simulink model "Gravity_Compensation"  (R2019a)
settings: Solver=FixedStepAuto  StartTime=0.0  StopTime=inf  RelTol=1e-3  EnableMultiTasking=on
libraries: eeGeneralControl x2, cm_custom x2
settings Model: SimulationMode=external  Creator=Ng Wee Shen  LastModifiedBy=rng
settings SolverCC: PositivePriorityOrder=on  AutoInsertRateTranBlk=on
settings DataIOCC: ReturnWorkspaceOutputs=off
settings OptimizationCC: EnhancedBackFolding=on  PassReuseOutputArgsAs=Individual arguments  MaxStackSize=64  OptimizeBlockOrder=speed  DifferentSizesBufferReuse=on
settings DebuggingCC: TimeAdjustmentMsg=warning  SingleTaskRateTransMsg=warning  ParameterTunabilityLossMsg=error  SFcnCompatibilityMsg=warning  ArithmeticOperatorsInVariantConditions=warning
settings HardwareCC: ProdBitPerPointer=32  ProdBitPerSizeT=32  ProdBitPerPtrDiffT=32  ProdLargestAtomicInteger=Long  ProdLargestAtomicFloat=Double  ProdWordSize=32  ProdHWDeviceType=ARM Compatible->ARM Cortex
settings SFSimCC: MATLABDynamicMemAlloc=off
settings RTWCC: SystemTargetFile=ert.tlc  HardwareBoard=Raspberry Pi  TLCOptions="-aInlineSetEventsForThisBaseRateFcn=TLC_FALSE -aSuppressMultiTaskScheduler=TLC_FALSE  -aRateBasedStepFcn=0"  TemplateMakefile=ert_default_tmf  Toolchain=GNU GCC Raspberry Pi  BuildConfiguration=Specify  IncludeHyperlinkInReport=on  TargetLang=C++
settings CodeAppCC: ForceParamTrailComments=on  IgnoreCustomStorageClasses=off  OperatorAnnotations=on  SimulinkDataObjDesc=on  SFDataObjDesc=on  InsertBlockDesc=on
settings ERTTargetCC: TargetLangStandard=C++03 (ISO)  SupportContinuousTime=on  SupportVariableSizeSignals=on  ExtMode=on  ExtModeMexArgs='192.168.0.173' 1 17725

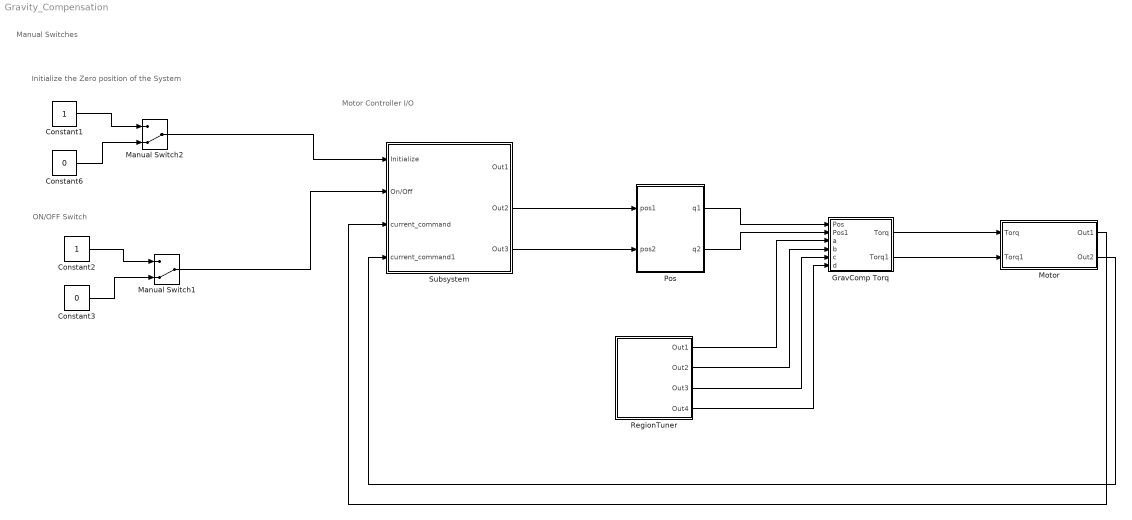
== system Gravity_Compensation ==
  note: Motor Controller I/O
  note: Manual Switches
  note: ON/OFF Switch
  note: Initialize the Zero position of the System
  Constant1 : Constant
  Constant2 : Constant
  Constant3 : Constant  Value=0
  Constant6 : Constant  Value=0
  GravComp Torq : MATLAB Function  TreatAsAtomicUnit=on
  Manual Switch1 : ManualSwitch  CurrentSetting=0
  Manual Switch2 : ManualSwitch  CurrentSetting=0
  Motor : Subsystem
  Pos : Subsystem
  RegionTuner : Subsystem
  Subsystem : Subsystem
  wires:
  Constant1/1 -> Manual Switch2/1
  Constant6/1 -> Manual Switch2/2
  Manual Switch2/1 -> Subsystem/1(Initialize)
  Subsystem/2(Out2) -> Pos/1(pos1)
  Subsystem/3(Out3) -> Pos/2(pos2)
  Constant2/1 -> Manual Switch1/1
  Constant3/1 -> Manual Switch1/2
  Manual Switch1/1 -> Subsystem/2(On/Off)
  GravComp Torq/1(Torq) -> Motor/1(Torq)
  GravComp Torq/2(Torq1) -> Motor/2(Torq1)
  Pos/1(q1) -> GravComp Torq/1(Pos)
  Pos/2(q2) -> GravComp Torq/2(Pos1)
  RegionTuner/1(Out1) -> GravComp Torq/3(a)
  RegionTuner/2(Out2) -> GravComp Torq/4(b)
  RegionTuner/3(Out3) -> GravComp Torq/5(c)
  RegionTuner/4(Out4) -> GravComp Torq/6(d)
  Motor/2(Out2) -> Subsystem/4(current_command1)
  Motor/1(Out1) -> Subsystem/3(current_command)

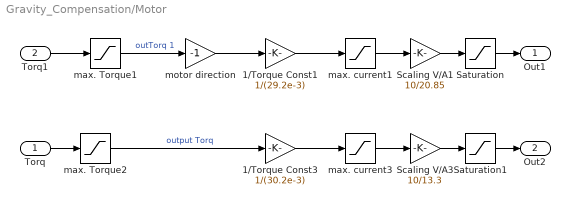
== system Gravity_Compensation/Motor ==
  Torq : Inport
  Torq1 : Inport  Port=2
  1/Torque Const1 : Gain  Gain=1/(29.2e-3)  OutDataTypeStr=Inherit: Same as input
  1/Torque Const3 : Gain  Gain=1/(30.2e-3)  OutDataTypeStr=Inherit: Same as input
  Saturation : Saturate  UpperLimit=9.95  LowerLimit=-9.95
  Saturation1 : Saturate  UpperLimit=9.95  LowerLimit=-9.95
  Scaling V/A1 : Gain  Gain=10/20.85  OutDataTypeStr=Inherit: Same as input
  Scaling V/A3 : Gain  Gain=10/13.3  OutDataTypeStr=Inherit: Same as input
  max. Torque1 : Saturate  UpperLimit=0.10  LowerLimit=-0.10
  max. Torque2 : Saturate  UpperLimit=0.05  LowerLimit=-0.05
  max. current1 : Saturate  UpperLimit=6  LowerLimit=-6
  max. current3 : Saturate  UpperLimit=6  LowerLimit=-6
  motor direction : Gain  Gain=-1  OutDataTypeStr=Inherit: Same as input
  Out1 : Outport
  Out2 : Outport  Port=2
  wires:
  max. current3/1 -> Scaling V/A3/1
  Scaling V/A3/1 -> Saturation1/1
  max. Torque2/1 -> 1/Torque Const3/1  "output Torq"
  Torq/1 -> max. Torque2/1
  1/Torque Const3/1 -> max. current3/1
  1/Torque Const1/1 -> max. current1/1
  max. current1/1 -> Scaling V/A1/1
  motor direction/1 -> 1/Torque Const1/1
  max. Torque1/1 -> motor direction/1  "outTorq 1"
  Scaling V/A1/1 -> Saturation/1
  Torq1/1 -> max. Torque1/1
  Saturation1/1 -> Out2/1
  Saturation/1 -> Out1/1

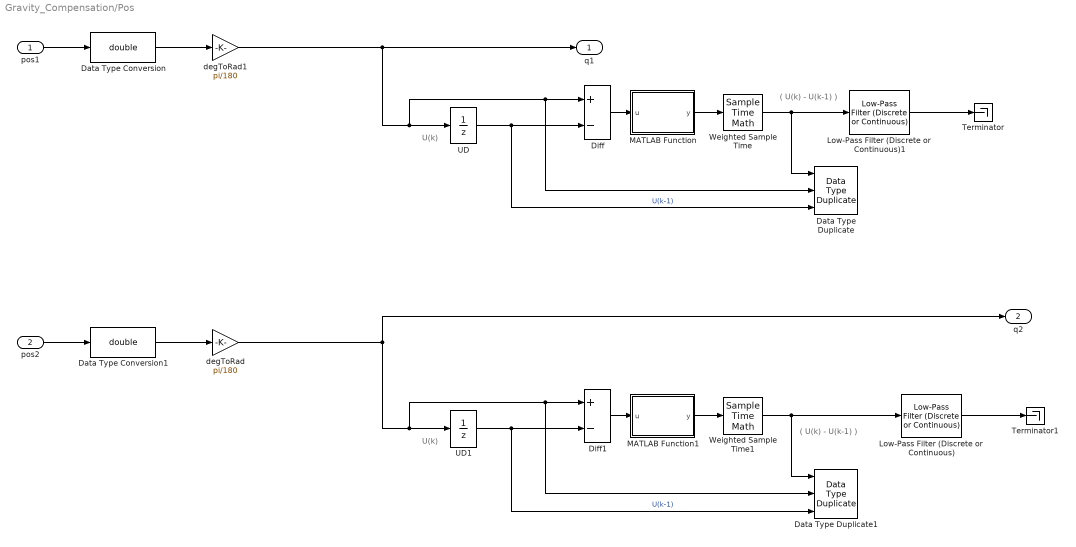
== system Gravity_Compensation/Pos ==
  note: ( U(k) - U(k-1) )
  note: U(k)
  note: U(k)
  note: ( U(k) - U(k-1) )
  pos1 : Inport
  pos2 : Inport  Port=2
  Data Type Duplicate : DataTypeDuplicate  DisableCoverage=on  NumInputPorts=3
  Data Type Duplicate1 : DataTypeDuplicate  DisableCoverage=on  NumInputPorts=3
  Data Type Conversion : DataTypeConversion  OutDataTypeStr=double
  Data Type Conversion1 : DataTypeConversion  OutDataTypeStr=double
  Diff : Sum  Description=Add in CPU  Inputs=+-
  Diff1 : Sum  Description=Add in CPU  Inputs=+-
  Low-Pass Filter (Discrete or Continuous) : eeGeneralControl/Low-Pass Filter (Discrete or Continuous)  K=1  T=0.01  B=inf  A=-inf  Ts=-1
      settings: SourceProductName=Simscape Electrical
  Low-Pass Filter (Discrete or Continuous)1 : eeGeneralControl/Low-Pass Filter (Discrete or Continuous)  K=1  T=0.01  B=inf  A=-inf  Ts=-1
      settings: SourceProductName=Simscape Electrical
  MATLAB Function : MATLAB Function  TreatAsAtomicUnit=on
  MATLAB Function1 : MATLAB Function  TreatAsAtomicUnit=on
  Terminator : Terminator
  Terminator1 : Terminator
  UD : UnitDelay  Description=Store in Global RAM  DisableCoverage=on  SampleTime=-1  HasFrameUpgradeWarning=on
  UD1 : UnitDelay  Description=Store in Global RAM  DisableCoverage=on  SampleTime=-1  HasFrameUpgradeWarning=on
  Weighted Sample Time : SampleTimeMath  TsampMathOp=/
  Weighted Sample Time1 : SampleTimeMath  TsampMathOp=/
  degToRad : Gain  Gain=pi/180
  degToRad1 : Gain  Gain=pi/180
  q1 : Outport
  q2 : Outport  Port=2
  wires:
  pos2/1 -> Data Type Conversion1/1
  pos1/1 -> Data Type Conversion/1
  Data Type Conversion1/1 -> degToRad/1
  Data Type Conversion/1 -> degToRad1/1
  Diff/1 -> MATLAB Function/1(u)
  UD/1 -> Diff/2, Data Type Duplicate/3  "U(k-1)"
  MATLAB Function/1(y) -> Weighted Sample Time/1
  Weighted Sample Time/1 -> Data Type Duplicate/1, Low-Pass Filter (Discrete or Continuous)1/1
  UD1/1 -> Diff1/2, Data Type Duplicate1/3  "U(k-1)"
  Diff1/1 -> MATLAB Function1/1(u)
  MATLAB Function1/1(y) -> Weighted Sample Time1/1
  Weighted Sample Time1/1 -> Data Type Duplicate1/1, Low-Pass Filter (Discrete or Continuous)/1
  degToRad1/1 -> q1/1, UD/1, Diff/1, Data Type Duplicate/2
  degToRad/1 -> q2/1, UD1/1, Diff1/1, Data Type Duplicate1/2
  Low-Pass Filter (Discrete or Continuous)1/1 -> Terminator/1
  Low-Pass Filter (Discrete or Continuous)/1 -> Terminator1/1

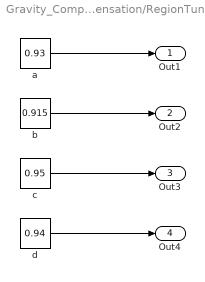
== system Gravity_Compensation/RegionTuner ==
  a : Constant  Value=0.93
  b : Constant  Value=0.915
  c : Constant  Value=0.95
  d : Constant  Value=0.94
  Out1 : Outport
  Out2 : Outport  Port=2
  Out3 : Outport  Port=3
  Out4 : Outport  Port=4
  wires:
  d/1 -> Out4/1
  b/1 -> Out2/1
  c/1 -> Out3/1
  a/1 -> Out1/1

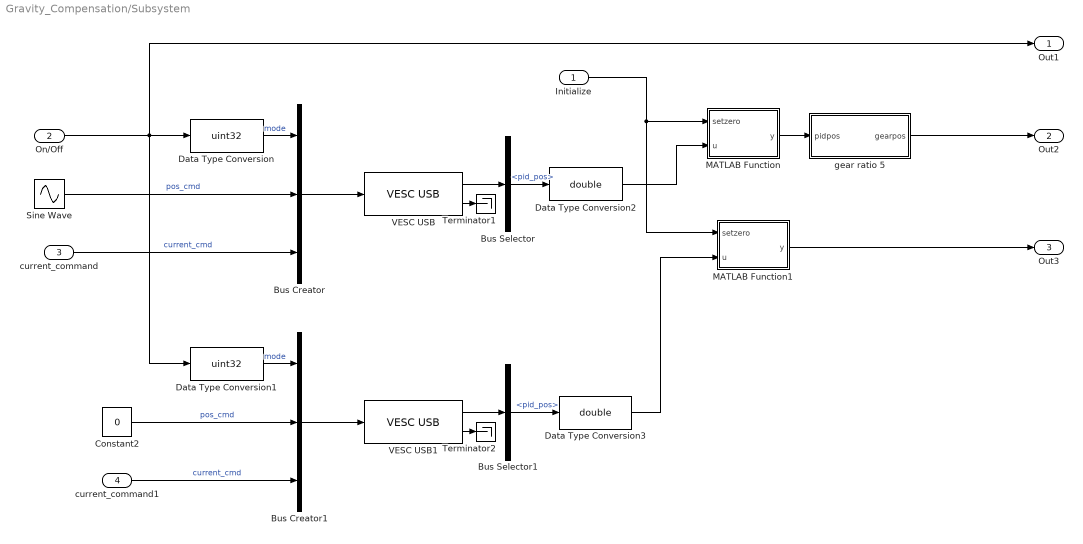
== system Gravity_Compensation/Subsystem ==
  Initialize : Inport
  On/Off : Inport  Port=2
  current_command : Inport  Port=3
  current_command1 : Inport  Port=4
  Bus Creator : BusCreator  Inputs=3
  Bus Creator1 : BusCreator  Inputs=3
  Bus Selector : BusSelector  OutputSignals=pid_pos
  Bus Selector1 : BusSelector  OutputSignals=pid_pos
  Constant2 : Constant  Value=0
  Data Type Conversion : DataTypeConversion  OutDataTypeStr=uint32
  Data Type Conversion1 : DataTypeConversion  OutDataTypeStr=uint32
  Data Type Conversion2 : DataTypeConversion  OutDataTypeStr=double
  Data Type Conversion3 : DataTypeConversion  OutDataTypeStr=double
  MATLAB Function : MATLAB Function  TreatAsAtomicUnit=on
  MATLAB Function1 : MATLAB Function  TreatAsAtomicUnit=on
  Sine Wave : Sin  Amplitude=150  Bias=10  SampleTime=0
  Terminator1 : Terminator
  Terminator2 : Terminator
  VESC USB : cm_custom/VESC USB  PAR_VESC_DEV='/dev/USB_VESC2'  POS_KP=0.03  POS_KI=0  POS_KD=0.0004  POS_KD_FIL=0.2  POS_DIV=1  CURR_MAX=6  CURR_MIN=-6  CURR_IN_MAX=99  CURR_IN_MIN=-60  CURR_ABS_MAX=130  PAR_SMPLT=0.001
      settings: SourceProductName=cm custom
  VESC USB1 : cm_custom/VESC USB  PAR_VESC_DEV='/dev/USB_VESC1'  POS_KP=0.001  POS_KI=0  POS_KD=0.001  POS_KD_FIL=0.2  POS_DIV=1  CURR_MAX=20  CURR_MIN=-20  CURR_IN_MAX=20  CURR_IN_MIN=-20  CURR_ABS_MAX=20  PAR_SMPLT=0.001
      settings: SourceProductName=cm custom
  gear ratio 5 : Subsystem
  Out1 : Outport
  Out2 : Outport  Port=2
  Out3 : Outport  Port=3
  wires:
  Bus Selector1/1 -> Data Type Conversion3/1  "<pid_pos>"
  Bus Creator1/1 -> VESC USB1/1
  Data Type Conversion3/1 -> MATLAB Function1/2(u)
  Data Type Conversion1/1 -> Bus Creator1/1  "mode"
  VESC USB/1 -> Bus Selector/1
  Sine Wave/1 -> Bus Creator/2  "pos_cmd"
  Bus Selector/1 -> Data Type Conversion2/1  "<pid_pos>"
  VESC USB1/2 -> Terminator2/1
  VESC USB/2 -> Terminator1/1
  Bus Creator/1 -> VESC USB/1
  Data Type Conversion2/1 -> MATLAB Function/2(u)
  Constant2/1 -> Bus Creator1/2  "pos_cmd"
  Initialize/1 -> MATLAB Function1/1(setzero), MATLAB Function/1(setzero)
  VESC USB1/1 -> Bus Selector1/1
  current_command1/1 -> Bus Creator1/3  "current_cmd"
  MATLAB Function/1(y) -> gear ratio 5/1(pidpos)
  Data Type Conversion/1 -> Bus Creator/1  "mode"
  gear ratio 5/1(gearpos) -> Out2/1
  MATLAB Function1/1(y) -> Out3/1
  On/Off/1 -> Data Type Conversion1/1, Out1/1, Data Type Conversion/1
  current_command/1 -> Bus Creator/3  "current_cmd"

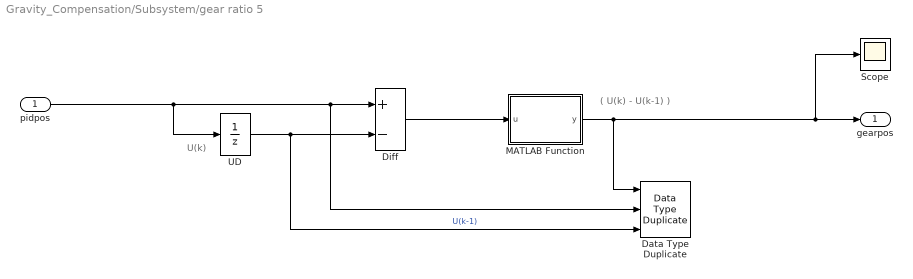
== system Gravity_Compensation/Subsystem/gear ratio 5 ==
  note: ( U(k) - U(k-1) )
  note: U(k)
  pidpos : Inport
  Data Type Duplicate : DataTypeDuplicate  DisableCoverage=on  NumInputPorts=3
  Diff : Sum  Description=Add in CPU  Inputs=+-
  MATLAB Function : MATLAB Function  TreatAsAtomicUnit=on
  Scope : Scope
  UD : UnitDelay  Description=Store in Global RAM  DisableCoverage=on  SampleTime=-1  HasFrameUpgradeWarning=on
  gearpos : Outport
  wires:
  UD/1 -> Diff/2, Data Type Duplicate/3  "U(k-1)"
  pidpos/1 -> UD/1, Diff/1, Data Type Duplicate/2
  MATLAB Function/1(y) -> Data Type Duplicate/1, Scope/1, gearpos/1
  Diff/1 -> MATLAB Function/1(u)

== matlab function Gravity_Compensation/Subsystem/MATLAB Function ==
  data: setzero input; u input; y output
function y = fcn(setzero,u)

persistent initpos
if isempty(initpos)
    initpos = 0;
end

if setzero
    initpos = u + 0;
end


y = u - initpos;
y = y - 360*floor(y/360);

== matlab function Gravity_Compensation/GravComp Torq ==
  data: Pos input; Pos1 input; Torq output; a input; Torq1 output; b input; c input; d input
function [Torq,Torq1] = fcn(Pos,Pos1,a,b,c,d)
%Pos=radians of joint 2 between -pi to pi
%Pos1=joint 1 between 0 to 2pi
Pos = Pos - 2*pi*floor((Pos + pi)./(2*pi));
Pos1 = Pos1 - 2*pi*floor(Pos1./(2*pi));
%G is the acquired parameter from sys id
%2.3 acquired from tuning 2nd joint only
G=[0.0291;0.0099*1.5];
PosM=[sin(Pos1) sin(Pos1+Pos); 0 sin(Pos1+Pos)];
Output=PosM*G;
%Torq=Joint 2 torq || Torq1=Joint 1 torq
Torq=Output(2);

%right and left area
if(abs(Pos1)<=pi/2)
    G=[0.0291*a;0.0099*0];
else
    if(abs(Pos1)>pi/2 &&abs(Pos1)<=pi)
        G=[0.0291*b;0.0099*0];
    else
        if(abs(Pos1)>pi &&abs(Pos1)<=((3/2)*pi))
        G=[0.0291*c;0.0099*0];
        else
        G=[0.0291*d;0.0099*0];
        end
    end
end
% G=[0.0291*0.92;0.0099*0];
PosM=[sin(Pos1) sin(Pos1+Pos); 0 sin(Pos1+Pos)];
Output=PosM*G;
Torq1=Output(1);

== matlab function Gravity_Compensation/Subsystem/MATLAB Function1 ==
  data: setzero input; u input; y output
function y = fcn(setzero,u)

persistent initpos
if isempty(initpos)
    initpos = 0;
end

if setzero
    initpos = u + 0;
end


y = u - initpos;
y = y - 360*floor(y/360);

== matlab function Gravity_Compensation/Pos/MATLAB Function ==
  data: u input; y output
function y = fcn(u)

u_rev = (u >= 0)*(2*pi - u) + (u < 0)*(2*pi + u);

if abs(u_rev) > abs(u)
   y = u;
else
   y = (u < 0)*u_rev - (u >= 0)*u_rev;
end

== matlab function Gravity_Compensation/Pos/MATLAB Function1 ==
  data: u input; y output
function y = fcn(u)

u_rev = (u >= 0)*(2*pi - u) + (u < 0)*(2*pi + u);

if abs(u_rev) > abs(u)
   y = u;
else
   y = (u < 0)*u_rev - (u >= 0)*u_rev;
end

== matlab function Gravity_Compensation/Subsystem/gear ratio 5/MATLAB Function ==
  data: u input; y output
function y = fcn(u)

persistent pos1
if isempty(pos1)
    pos1 = 0;
end

u_rev = (u >= 0)*(360 - u) + (u < 0)*(360 + u);
if abs(u_rev) < abs(u)
   u = (u < 0)*u_rev - (u >= 0)*u_rev;
end

u = u/5;
pos1 = pos1 + u;
pos1 = mod((pos1),360);
y = pos1;

end
